simulink model "d2kontur_d2"  (R2014b)
settings: Solver=ode3  SolverMode=SingleTasking  StartTime=0.0  StopTime=10.0  RelTol=1e-3
PreLoadFcn:
  | waijung.modelPreload; % Required for working with Waijung Blockset. Do not remove.
undefined symbols (not defined in the file): FiO2, HCLK, HSEOSC, Link, LQFP100, ST, STM32F407VE
libraries: simulink_extras x8, stm32f4_io_lib x2, stm32f4_adc_lib x1, stm32f4_device_config_lib x1
(part 2 of 2)

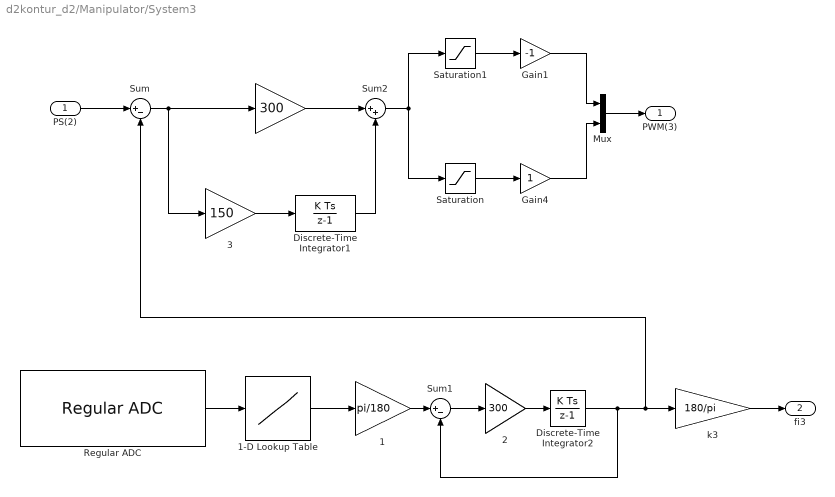
== system d2kontur_d2/Manipulator/System3 ==
  PS(2) : Inport
  " " : Gain  Gain=300
  " 1" : Gain  Gain=pi/180
  " 2" : Gain  Gain=300
  " 3" : Gain  Gain=150
  1-D Lookup Table : Lookup_n-D  NumberOfTableDimensions=1  BreakpointsForDimension1=[0 645 1470 2290 3115]  Table=[-180 -90 0 90 180]  InternalRulePriority=Speed  RndMeth=Simplest  InputSameDT=on
  Discrete-Time Integrator1 : DiscreteIntegrator  SampleTime=0.001  LimitOutput=on  UpperSaturationLimit=50  LowerSaturationLimit=-50
  Discrete-Time Integrator2 : DiscreteIntegrator  SampleTime=0.001
  Gain1 : Gain  Gain=-1  OutDataTypeStr=double
  Gain4 : Gain  OutDataTypeStr=double
  Mux : Mux  Inputs=2
  Regular ADC : stm32f4_adc_lib/Regular ADC  adcmodule=1  outputdatatype=Double  prescaler=2  prescalerstr=ADC_Prescaler_Div2  chsamplingtime=Auto  chsamplingtimestr=ADC_SampleTime_480Cycles  read_an0=off  read_an1=off  read_an2=off  read_an3=off  read_an4=off  read_an5=off  read_an6=off  read_an7=off  read_an8=off  read_an9=off  read_an10=off  read_an11=on  read_an12=off  read_an13=off  read_an14=off  read_an15=off  read_an16=off  read_an17=off  read_an18=off  pinstr=GPIO_Pin_11  usedpinarray="[0  0  0  0  0  0  0  0  0  0  0  1  0  0  0  0  0  0  0]"  usedportidarray=[2]  usedpinidarray=[1]  usedpinidcount=1  sampletime=0.001  blockid=ManipulatorSystem3RegularADC  enablecustomportlabel=off  cinputportlabel=0  coutputportlabel=Out1, Out2
  Saturation : Saturate  UpperLimit=80  LowerLimit=0  SampleTime=0.001
  Saturation1 : Saturate  UpperLimit=0  LowerLimit=-80  SampleTime=0.001
  Sum : Sum  Inputs=|+-
  Sum1 : Sum  Inputs=|+-
  Sum2 : Sum  Inputs=|++
  k3 : Gain  Gain=180/pi
  PWM(3) : Outport
  fi3 : Outport  Port=2
  wires:
  Saturation1/1 -> Gain1/1
  Saturation/1 -> Gain4/1
  PS(2)/1 -> Sum/1
  Gain1/1 -> Mux/1
  Gain4/1 -> Mux/2
  1-D Lookup Table/1 -> " 1"/1
  Mux/1 -> PWM(3)/1
  Sum2/1 -> Saturation/1, Saturation1/1
  Sum/1 -> " 3"/1, " "/1
  " 1"/1 -> Sum1/1
  Discrete-Time Integrator2/1 -> k3/1, Sum/2, Sum1/2
  Discrete-Time Integrator1/1 -> Sum2/2
  Regular ADC/1 -> 1-D Lookup Table/1
  " "/1 -> Sum2/1
  " 3"/1 -> Discrete-Time Integrator1/1
  Sum1/1 -> " 2"/1
  " 2"/1 -> Discrete-Time Integrator2/1
  k3/1 -> fi3/1

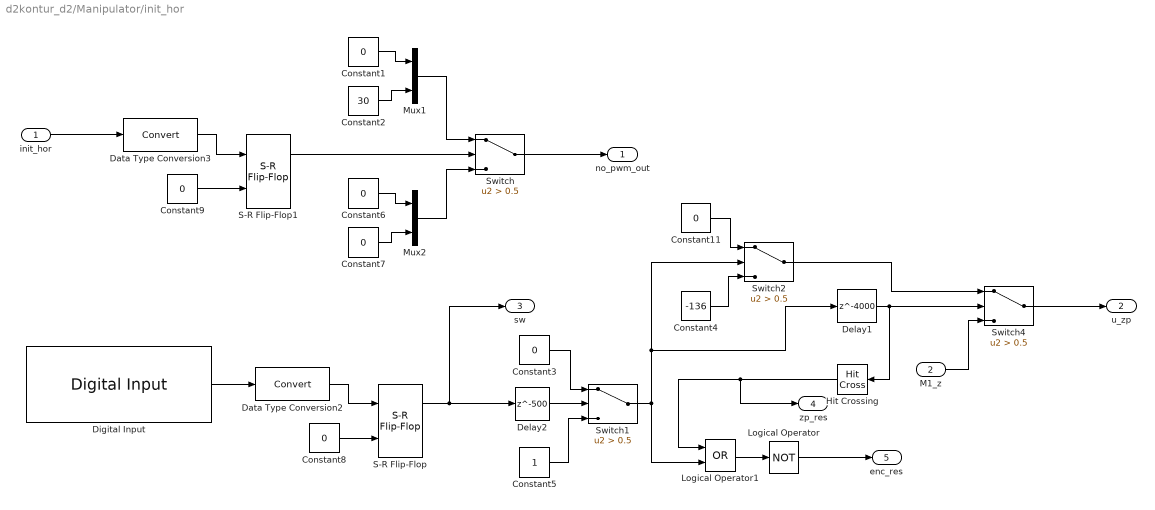
== system d2kontur_d2/Manipulator/init_hor ==
  init_hor : Inport
  M1_z : Inport  Port=2
  Constant{1,3,6..7,11} (5 alike) : Constant  Value=0
  Constant2 : Constant  Value=30
  Constant4 : Constant  Value=-136
  Constant5 : Constant
  Constant8 : Constant  Value=0  OutDataTypeStr=boolean
  Constant9 : Constant  Value=0  OutDataTypeStr=boolean
  Data Type Conversion2 : DataTypeConversion
  Data Type Conversion3 : DataTypeConversion
  Delay1 : Delay  DelayLength=4000
  Delay2 : Delay  DelayLength=500
  Digital Input : stm32f4_io_lib/Digital Input  port=B  speed=100  porttype=None  porttypestr=NOPULL  use_pin0=off  use_pin1=off  use_pin2=off  use_pin3=on  use_pin4=off  use_pin5=off  use_pin6=off  use_pin7=off  use_pin8=off  use_pin9=off  use_pin10=off  use_pin11=off  use_pin12=off  use_pin13=off  use_pin14=off  use_pin15=off  pinstr=GPIO_Pin_3  usedpinarray="[0  0  0  1  0  0  0  0  0  0  0  0  0  0  0  0]"  bitbandingstr="#define Manipulatorinit_horDigitalInput_B3 Peripheral_BB(GPIOB->IDR, 3)  /* Output pin */"  sampletime=0.001  sampletimestr=-1  blockid=Manipulatorinit_horDigitalInput  enablecustomportlabel=off  glabalinit=off  cinputportlabel=In1, In2  coutputportlabel=Out1, Out2
  Hit Crossing : HitCross  HitCrossingOffset=0.5  HitCrossingDirection=falling
  Logical Operator : Logic  Operator=NOT  AllPortsSameDT=off  OutDataTypeStr=boolean
  Logical Operator1 : Logic  Operator=OR  AllPortsSameDT=off  OutDataTypeStr=boolean
  Mux1 : Mux  Inputs=2
  Mux2 : Mux  Inputs=2
  S-R Flip-Flop : simulink_extras/Flip Flops/S-R Flip-Flop  initial_condition=0
  S-R Flip-Flop1 : simulink_extras/Flip Flops/S-R Flip-Flop  initial_condition=0
  Switch{,1..2,4} (4 alike) : Switch  Criteria=u2 > Threshold  Threshold=0.5
  no_pwm_out : Outport
  u_zp : Outport  Port=2
  sw : Outport  Port=3
  zp_res : Outport  Port=4
  enc_res : Outport  Port=5
  wires:
  init_hor/1 -> Data Type Conversion3/1
  Constant5/1 -> Switch1/3
  S-R Flip-Flop1/1 -> Switch/2
  Switch2/1 -> Switch4/1
  Data Type Conversion3/1 -> S-R Flip-Flop1/1
  Constant9/1 -> S-R Flip-Flop1/2
  S-R Flip-Flop/1 -> sw/1, Delay2/1
  Switch4/1 -> u_zp/1
  Switch/1 -> no_pwm_out/1
  Digital Input/1 -> Data Type Conversion2/1
  Constant8/1 -> S-R Flip-Flop/2
  Data Type Conversion2/1 -> S-R Flip-Flop/1
  Mux2/1 -> Switch/3
  Mux1/1 -> Switch/1
  Hit Crossing/1 -> zp_res/1, Logical Operator1/1
  M1_z/1 -> Switch4/3
  Logical Operator/1 -> enc_res/1
  Delay1/1 -> Switch4/2, Hit Crossing/1
  Switch1/1 -> Logical Operator1/2, Delay1/1, Switch2/2
  Delay2/1 -> Switch1/2
  Logical Operator1/1 -> Logical Operator/1
  Constant1/1 -> Mux1/1
  Constant2/1 -> Mux1/2
  Constant6/1 -> Mux2/1
  Constant7/1 -> Mux2/2
  Constant3/1 -> Switch1/1
  Constant4/1 -> Switch2/3
  Constant11/1 -> Switch2/1

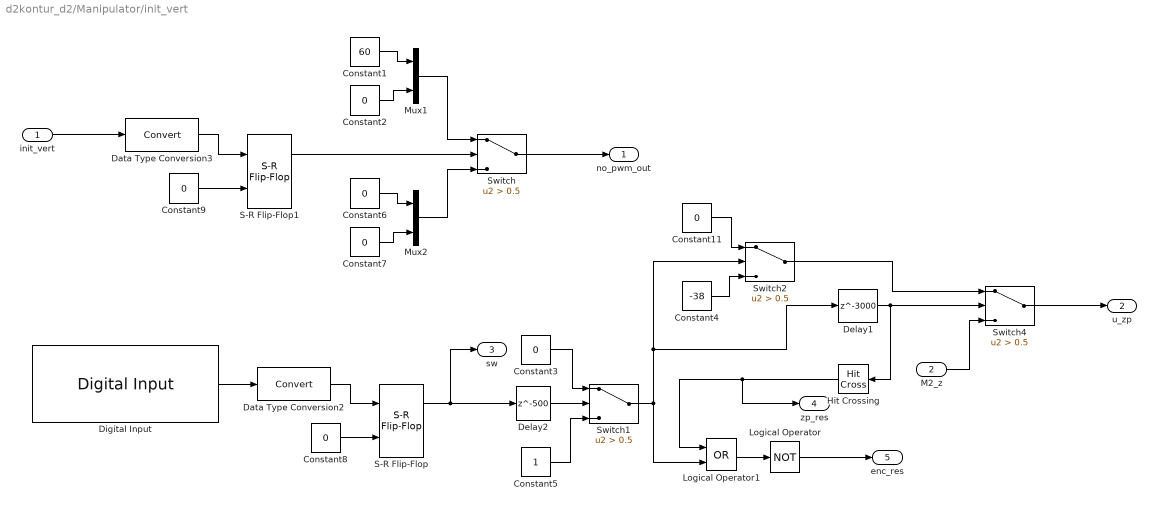
== system d2kontur_d2/Manipulator/init_vert ==
  init_vert : Inport
  M2_z : Inport  Port=2
  Constant1 : Constant  Value=60
  Constant{2..3,6..7,11} (5 alike) : Constant  Value=0
  Constant4 : Constant  Value=-38
  Constant5 : Constant
  Constant8 : Constant  Value=0  OutDataTypeStr=boolean
  Constant9 : Constant  Value=0  OutDataTypeStr=boolean
  Data Type Conversion2 : DataTypeConversion
  Data Type Conversion3 : DataTypeConversion
  Delay1 : Delay  DelayLength=3000
  Delay2 : Delay  DelayLength=500
  Digital Input : stm32f4_io_lib/Digital Input  port=D  speed=100  porttype=None  porttypestr=NOPULL  use_pin0=on  use_pin1=off  use_pin2=off  use_pin3=off  use_pin4=off  use_pin5=off  use_pin6=off  use_pin7=off  use_pin8=off  use_pin9=off  use_pin10=off  use_pin11=off  use_pin12=off  use_pin13=off  use_pin14=off  use_pin15=off  pinstr=GPIO_Pin_0  usedpinarray="[1  0  0  0  0  0  0  0  0  0  0  0  0  0  0  0]"  bitbandingstr="#define Manipulatorinit_vertDigitalInput_D0 Peripheral_BB(GPIOD->IDR, 0)  /* Output pin */"  sampletime=0.001  sampletimestr=-1  blockid=Manipulatorinit_vertDigitalInput  enablecustomportlabel=off  glabalinit=off  cinputportlabel=In1, In2  coutputportlabel=Out1, Out2
  Hit Crossing : HitCross  HitCrossingOffset=0.5  HitCrossingDirection=falling
  Logical Operator : Logic  Operator=NOT  AllPortsSameDT=off  OutDataTypeStr=boolean
  Logical Operator1 : Logic  Operator=OR  AllPortsSameDT=off  OutDataTypeStr=boolean
  Mux1 : Mux  Inputs=2
  Mux2 : Mux  Inputs=2
  S-R Flip-Flop : simulink_extras/Flip Flops/S-R Flip-Flop  initial_condition=0
  S-R Flip-Flop1 : simulink_extras/Flip Flops/S-R Flip-Flop  initial_condition=0
  Switch{,1..2,4} (4 alike) : Switch  Criteria=u2 > Threshold  Threshold=0.5
  no_pwm_out : Outport
  u_zp : Outport  Port=2
  sw : Outport  Port=3
  zp_res : Outport  Port=4
  enc_res : Outport  Port=5
  wires:
  Constant11/1 -> Switch2/1
  Constant3/1 -> Switch1/1
  Constant7/1 -> Mux2/2
  Constant6/1 -> Mux2/1
  Constant2/1 -> Mux1/2
  Constant1/1 -> Mux1/1
  Logical Operator1/1 -> Logical Operator/1
  Delay2/1 -> Switch1/2
  Switch1/1 -> Switch2/2, Delay1/1, Logical Operator1/2
  Delay1/1 -> Hit Crossing/1, Switch4/2
  Logical Operator/1 -> enc_res/1
  M2_z/1 -> Switch4/3
  Hit Crossing/1 -> Logical Operator1/1, zp_res/1
  Mux1/1 -> Switch/1
  Mux2/1 -> Switch/3
  Data Type Conversion2/1 -> S-R Flip-Flop/1
  Constant8/1 -> S-R Flip-Flop/2
  Digital Input/1 -> Data Type Conversion2/1
  Switch/1 -> no_pwm_out/1
  Switch4/1 -> u_zp/1
  S-R Flip-Flop/1 -> Delay2/1, sw/1
  Constant9/1 -> S-R Flip-Flop1/2
  Data Type Conversion3/1 -> S-R Flip-Flop1/1
  Switch2/1 -> Switch4/1
  S-R Flip-Flop1/1 -> Switch/2
  Constant5/1 -> Switch1/3
  init_vert/1 -> Data Type Conversion3/1
  Constant4/1 -> Switch2/3

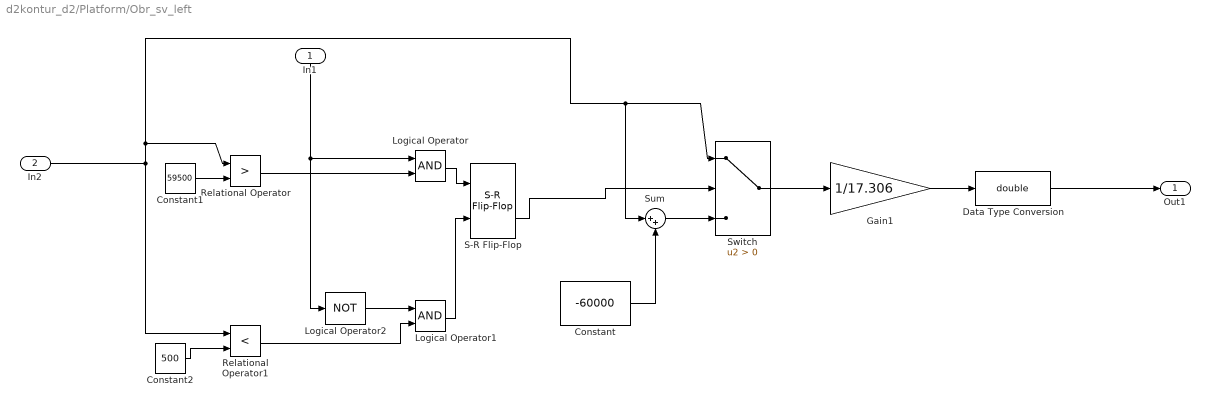
== system d2kontur_d2/Platform/Obr_sv_left ==
  In1 : Inport
  In2 : Inport  Port=2
  Constant : Constant  Value=-60000
  Constant1 : Constant  Value=59500
  Constant2 : Constant  Value=500
  Data Type Conversion : DataTypeConversion  OutDataTypeStr=double
  Gain1 : Gain  Gain=1/17.306
  Logical Operator : Logic  AllPortsSameDT=off  OutDataTypeStr=boolean
  Logical Operator1 : Logic  AllPortsSameDT=off  OutDataTypeStr=boolean
  Logical Operator2 : Logic  Operator=NOT  AllPortsSameDT=off  OutDataTypeStr=boolean
  Relational Operator : RelationalOperator  Operator=>  OutDataTypeStr=boolean
  Relational Operator1 : RelationalOperator  Operator=<  OutDataTypeStr=boolean
  S-R Flip-Flop : simulink_extras/Flip Flops/S-R Flip-Flop  initial_condition=0
  Sum : Sum  Inputs=|++
  Switch : Switch  Criteria=u2 > Threshold
  Out1 : Outport
  wires:
  Constant/1 -> Sum/2
  Relational Operator/1 -> Logical Operator/2
  Logical Operator/1 -> S-R Flip-Flop/1
  Relational Operator1/1 -> Logical Operator1/2
  Logical Operator1/1 -> S-R Flip-Flop/2
  In2/1 -> Switch/1, Sum/1, Relational Operator/1, Relational Operator1/1
  Sum/1 -> Switch/3
  Constant1/1 -> Relational Operator/2
  Constant2/1 -> Relational Operator1/2
  S-R Flip-Flop/2 -> Switch/2
  In1/1 -> Logical Operator/1, Logical Operator2/1
  Logical Operator2/1 -> Logical Operator1/1
  Gain1/1 -> Data Type Conversion/1
  Switch/1 -> Gain1/1
  Data Type Conversion/1 -> Out1/1

== system d2kontur_d2/Platform/Obr_sv_right ==
  In1 : Inport
  In2 : Inport  Port=2
  Constant : Constant  Value=-60000
  Constant1 : Constant  Value=59500
  Constant2 : Constant  Value=500
  Data Type Conversion : DataTypeConversion  OutDataTypeStr=double
  Gain1 : Gain  Gain=1/17.306
  Logical Operator : Logic  AllPortsSameDT=off  OutDataTypeStr=boolean
  Logical Operator1 : Logic  AllPortsSameDT=off  OutDataTypeStr=boolean
  Logical Operator2 : Logic  Operator=NOT  AllPortsSameDT=off  OutDataTypeStr=boolean
  Relational Operator : RelationalOperator  Operator=>  OutDataTypeStr=boolean
  Relational Operator1 : RelationalOperator  Operator=<  OutDataTypeStr=boolean
  S-R Flip-Flop : simulink_extras/Flip Flops/S-R Flip-Flop  initial_condition=0
  Sum : Sum  Inputs=|++
  Switch : Switch  Criteria=u2 > Threshold
  Out1 : Outport
  wires:
  Logical Operator2/1 -> Logical Operator1/1
  In1/1 -> Logical Operator2/1, Logical Operator/1
  S-R Flip-Flop/2 -> Switch/2
  Constant2/1 -> Relational Operator1/2
  Constant1/1 -> Relational Operator/2
  Sum/1 -> Switch/3
  In2/1 -> Relational Operator1/1, Relational Operator/1, Sum/1, Switch/1
  Logical Operator1/1 -> S-R Flip-Flop/2
  Relational Operator1/1 -> Logical Operator1/2
  Logical Operator/1 -> S-R Flip-Flop/1
  Relational Operator/1 -> Logical Operator/2
  Constant/1 -> Sum/2
  Gain1/1 -> Data Type Conversion/1
  Switch/1 -> Gain1/1
  Data Type Conversion/1 -> Out1/1

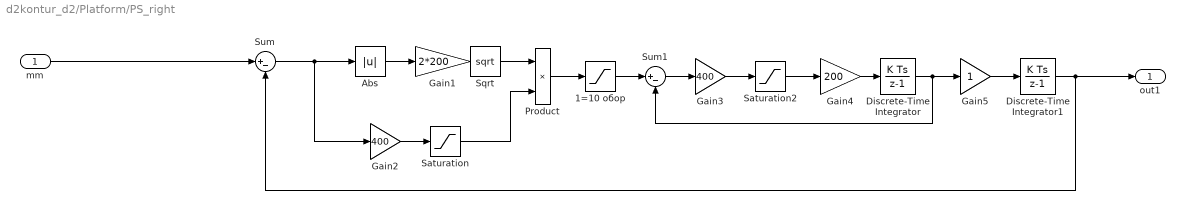
== system d2kontur_d2/Platform/PS_right  ==
  mm : Inport
  1=10 обор : Saturate  UpperLimit=200  LowerLimit=-200
  Abs : Abs
  Discrete-Time Integrator : DiscreteIntegrator  SampleTime=0.001
  Discrete-Time Integrator1 : DiscreteIntegrator  SampleTime=0.001
  Gain1 : Gain  Gain=2*200
  Gain2 : Gain  Gain=400
  Gain3 : Gain  Gain=400
  Gain4 : Gain  Gain=200
  Gain5 : Gain
  Product : Product
  Saturation : Saturate  UpperLimit=1  LowerLimit=-1
  Saturation2 : Saturate  UpperLimit=1  LowerLimit=-1
  Sqrt : Sqrt  SaturateOnIntegerOverflow=on
  Sum : Sum  Inputs=|+-
  Sum1 : Sum  Inputs=|+-
  "out1 " : Outport
  wires:
  mm/1 -> Sum/1
  Abs/1 -> Gain1/1
  Sum/1 -> Gain2/1, Abs/1
  Gain1/1 -> Sqrt/1
  Sqrt/1 -> Product/1
  Gain3/1 -> Saturation2/1
  1=10 обор/1 -> Sum1/1
  Saturation/1 -> Product/2
  Discrete-Time Integrator1/1 -> "out1 "/1, Sum/2
  Product/1 -> 1=10 обор/1
  Gain5/1 -> Discrete-Time Integrator1/1
  Sum1/1 -> Gain3/1
  Gain2/1 -> Saturation/1
  Discrete-Time Integrator/1 -> Gain5/1, Sum1/2
  Saturation2/1 -> Gain4/1
  Gain4/1 -> Discrete-Time Integrator/1

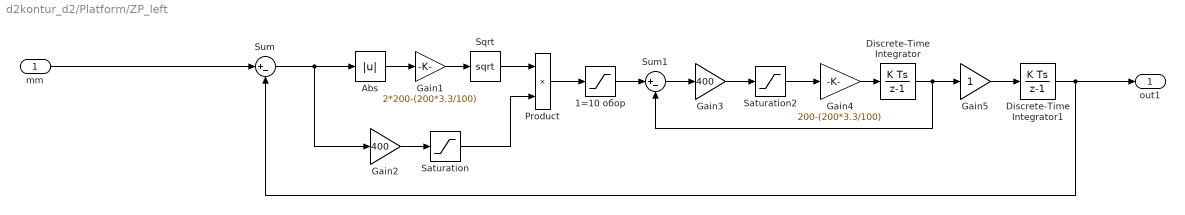
== system d2kontur_d2/Platform/ZP_left ==
  mm : Inport
  1=10 обор : Saturate  UpperLimit=200-(200*3.3/100)  LowerLimit=-(200-(200*3.3/100))
  Abs : Abs
  Discrete-Time Integrator : DiscreteIntegrator  SampleTime=0.001
  Discrete-Time Integrator1 : DiscreteIntegrator  SampleTime=0.001
  Gain1 : Gain  Gain=2*200-(200*3.3/100)
  Gain2 : Gain  Gain=400
  Gain3 : Gain  Gain=400
  Gain4 : Gain  Gain=200-(200*3.3/100)
  Gain5 : Gain
  Product : Product
  Saturation : Saturate  UpperLimit=1  LowerLimit=-1
  Saturation2 : Saturate  UpperLimit=1  LowerLimit=-1
  Sqrt : Sqrt  SaturateOnIntegerOverflow=on
  Sum : Sum  Inputs=|+-
  Sum1 : Sum  Inputs=|+-
  "out1 " : Outport
  wires:
  Gain4/1 -> Discrete-Time Integrator/1
  Saturation2/1 -> Gain4/1
  Discrete-Time Integrator/1 -> Sum1/2, Gain5/1
  Gain2/1 -> Saturation/1
  Sum1/1 -> Gain3/1
  Gain5/1 -> Discrete-Time Integrator1/1
  Product/1 -> 1=10 обор/1
  Discrete-Time Integrator1/1 -> Sum/2, "out1 "/1
  Saturation/1 -> Product/2
  1=10 обор/1 -> Sum1/1
  Gain3/1 -> Saturation2/1
  Sqrt/1 -> Product/1
  Gain1/1 -> Sqrt/1
  Sum/1 -> Abs/1, Gain2/1
  Abs/1 -> Gain1/1
  mm/1 -> Sum/1

== system d2kontur_d2/Platform/left ==
  Zadanie : Inport
  Obr_sv : Inport  Port=2
  Gain1 : Gain  Gain=-1
  Gain5 : Gain  Gain=10
  Saturation1 : Saturate  UpperLimit=100  LowerLimit=0
  Saturation4 : Saturate  UpperLimit=0  LowerLimit=-100
  Sum : Sum  Inputs=|+-
  Out1 : Outport
  Out2 : Outport  Port=2
  wires:
  Gain1/1 -> Out1/1
  Saturation1/1 -> Out2/1
  Saturation4/1 -> Gain1/1
  Zadanie/1 -> Sum/1
  Obr_sv/1 -> Sum/2
  Gain5/1 -> Saturation4/1, Saturation1/1
  Sum/1 -> Gain5/1

== system d2kontur_d2/Platform/right ==
  Zadanie : Inport
  Obr_sv : Inport  Port=2
  Gain1 : Gain  Gain=-1
  Gain4 : Gain  Gain=-1
  Gain5 : Gain  Gain=10
  Saturation1 : Saturate  UpperLimit=100  LowerLimit=0
  Saturation4 : Saturate  UpperLimit=0  LowerLimit=-100
  Sum : Sum  Inputs=|+-
  Out1 : Outport
  Out2 : Outport  Port=2
  wires:
  Obr_sv/1 -> Sum/2
  Zadanie/1 -> Gain4/1
  Saturation4/1 -> Gain1/1
  Saturation1/1 -> Out2/1
  Gain1/1 -> Out1/1
  Gain5/1 -> Saturation4/1, Saturation1/1
  Sum/1 -> Gain5/1
  Gain4/1 -> Sum/1

== system d2kontur_d2/Signal_generation/SW1 ==
  ind2 : Inport
  ind1 : Inport  Port=2
  sravn : Inport  Port=3
  "Obr_sv " : Inport  Port=4
  Relational Operator : RelationalOperator  Operator===  OutDataTypeStr=boolean
  Switch3 : Switch  Criteria=u2 > Threshold  Threshold=0.5
  M1 : Outport
  wires:
  ind1/1 -> Relational Operator/1
  Switch3/1 -> M1/1
  sravn/1 -> Relational Operator/2
  "Obr_sv "/1 -> Switch3/3
  ind2/1 -> Switch3/1
  Relational Operator/1 -> Switch3/2

== system d2kontur_d2/Signal_generation/SW2 ==
  ind2 : Inport
  ind1 : Inport  Port=2
  sravn : Inport  Port=3
  "Obr_sv " : Inport  Port=4
  Relational Operator : RelationalOperator  Operator===  OutDataTypeStr=boolean
  Switch3 : Switch  Criteria=u2 > Threshold  Threshold=0.5
  M2 : Outport
  wires:
  Relational Operator/1 -> Switch3/2
  ind2/1 -> Switch3/1
  "Obr_sv "/1 -> Switch3/3
  sravn/1 -> Relational Operator/2
  Switch3/1 -> M2/1
  ind1/1 -> Relational Operator/1

== system d2kontur_d2/Signal_generation/SW3 ==
  ind2 : Inport
  ind1 : Inport  Port=2
  sravn : Inport  Port=3
  "Obr_sv " : Inport  Port=4
  Relational Operator : RelationalOperator  Operator===  OutDataTypeStr=boolean
  Switch3 : Switch  Criteria=u2 > Threshold  Threshold=0.5
  M3 : Outport
  wires:
  ind1/1 -> Relational Operator/1
  Switch3/1 -> M3/1
  sravn/1 -> Relational Operator/2
  "Obr_sv "/1 -> Switch3/3
  ind2/1 -> Switch3/1
  Relational Operator/1 -> Switch3/2

== system d2kontur_d2/Signal_generation/SWT ==
  ind2 : Inport
  ind1 : Inport  Port=2
  sravn : Inport  Port=3
  "Obr_sv " : Inport  Port=4
  Relational Operator : RelationalOperator  Operator===  OutDataTypeStr=boolean
  Switch3 : Switch  Criteria=u2 > Threshold  Threshold=0.5
  Platform : Outport
  wires:
  Relational Operator/1 -> Switch3/2
  ind2/1 -> Switch3/1
  "Obr_sv "/1 -> Switch3/3
  sravn/1 -> Relational Operator/2
  Switch3/1 -> Platform/1
  ind1/1 -> Relational Operator/1

== system d2kontur_d2/Manipulator/System1/PositionFeedback ==
  Enable : EnablePort
  Data Type Conversion1 : DataTypeConversion  OutDataTypeStr=double
  Data Type Conversion2 : DataTypeConversion  OutDataTypeStr=double
  Encoder Read1 : S-Function  FunctionName=stm32f4_encoderread  Parameters=sampletime,sampletimestr,blockid,timer,apb,portstr,pinstr,pinmat,chmat,filterstr,filter,factor,rstcnt,ppr  EnableBusSupport=off  mask(stm32f4_encoderread){timer=3, ch1=A6, ch2=B5, ppr=10000, rstcnt=off, filterstr=No filter; sampling is done at fDTS, sampletime=0.001, sampletimestr=-1, blockid=ManipulatorSystem1PositionFeedbackEncoderRead1, absresetinput=off, portpinstr=A6,B5, portstr=["A","B"], pinstr=["GPIO_Pin_6","GPIO_Pin_5"], pinmat=[1 6;1 5], chmat=[1  2], apb=1, filter=0, factor=4}
      mask prompts: ch1 "Channel A Input Pin"; ch2 "Channel B Input Pin"; ppr "PPR (Number of pulses generated per revolution)"; rstcnt "Reset counter after every counter read"; filterstr "Built-in Input Capture Filter"; sampletime "Sample time (sec)"; sampletimestr "Compiled sample time (sec) in string"; absresetinput "Enable absolute position reset input signal"; portpinstr "Port pin string"; portstr "Port string"; pinstr "Pin string"; pinmat "Pin matrix"; chmat "Channel order"; filter "Filter ID"
      mask help:
      | The output Direction (uint32) is the direction of rotation either 0 or 1.
      |
      | The output Position (count) (uint32) is the count of number of edges of the encoder output signals from either channel A and B. The decoder is set to count at every rising and falling edge of both channel A and B (4x) or (x2) for one channel. For example, if an encoder has 180 pulses per revolution (PPS) and two channels are selected, the maximum count is 720 per revolution (4x180 = 720), i.e. from 0 to 719.
      mask init:
      | stm32f4_encoderread_callback('init');
      mask Help: web(fullfile(waijungdocroot,'stm32f4_encoderread.htm'),'-browser')
      mask TypeOptions timer: 1 | 2 | 3 | 4 | 5 | 8
      mask Callback timer: stm32f4_encoderread_callback('timer');
      mask TypeOptions ch1: Not available - Do not use | A6 | C6 | B4
      mask Callback ch1: stm32f4_encoderread_callback('chA');
      mask TypeOptions ch2: Not available - Do not use | A7 | C7 | B5
      mask Callback ch2: stm32f4_encoderread_callback('chB');
      mask Callback ppr: stm32f4_encoderread_callback('ppr');
      mask Callback rstcnt: stm32f4_encoderread_callback('rstcnt');
      mask TypeOptions filterstr: No filter; sampling is done at fDTS | fSAMPLING=fCK_INT; N=2 | fSAMPLING=fCK_INT; N=4 | fSAMPLING=fCK_INT; N=8 | fSAMPLING=fDTS/2; N=6 | fSAMPLING=fDTS/2; N=8 | fSAMPLING=fDTS/4; N=6 | fSAMPLING=fDTS/4; N=8 | fSAMPLING=fDTS/8; N=6 | fSAMPLING=fDTS/8; N=8 | fSAMPLING=fDTS/16; N=5 | fSAMPLING=fDTS/16; N=6 | fSAMPLING=fDTS/16; N=8 | fSAMPLING=fDTS/32; N=5 | fSAMPLING=fDTS/32; N=6 | fSAMPLING=fDTS/32; N=8
      mask Callback filterstr: stm32f4_encoderread_callback('filterstr');
      mask Callback sampletimestr: stm32f4_encoderread_callback('sampletimestr');
      mask Callback blockid: stm32f4_encoderread_callback('blockid');
      mask Display: text(0.05, 0.5, 'Timer: 3\nInput pins [CH_A, CH_B]: [A6,B5]\nRST Counter: No\nTs (sec): -1','ver','middle','hor','left');port_label('output', 1, 'Direction');port_label('output', 2, 'Position (count)')
  To_Bipolar : Subsystem
  To_radians : Gain  Gain=pi/48.8/180
  ps_rad : Outport
  wires:
  To_Bipolar/1(Out1) -> To_radians/1
  Encoder Read1/2 -> Data Type Conversion1/1
  Encoder Read1/1 -> Data Type Conversion2/1
  Data Type Conversion2/1 -> To_Bipolar/1(In1)
  To_radians/1 -> ps_rad/1
  Data Type Conversion1/1 -> To_Bipolar/2(In2)

== system d2kontur_d2/Manipulator/System2/Subsystem ==
  Enable : EnablePort
  Data Type Conversion1 : DataTypeConversion  OutDataTypeStr=double
  Data Type Conversion2 : DataTypeConversion  OutDataTypeStr=double
  Encoder Read : S-Function  FunctionName=stm32f4_encoderread  Parameters=sampletime,sampletimestr,blockid,timer,apb,portstr,pinstr,pinmat,chmat,filterstr,filter,factor,rstcnt,ppr  EnableBusSupport=off  mask(stm32f4_encoderread){timer=4, ch1=B6, ch2=B7, ppr=27034, rstcnt=off, filterstr=No filter; sampling is done at fDTS, sampletime=0.001, sampletimestr=-1, blockid=ManipulatorSystem2SubsystemEncoderRead, absresetinput=off, portpinstr=B6,B7, portstr=["B"], pinstr=["GPIO_Pin_6 | GPIO_Pin_7"], pinmat=[2 6 7], chmat=[1  2], apb=1, filter=0, factor=4}
      mask prompts: ch1 "Channel A Input Pin"; ch2 "Channel B Input Pin"; ppr "PPR (Number of pulses generated per revolution)"; rstcnt "Reset counter after every counter read"; filterstr "Built-in Input Capture Filter"; sampletime "Sample time (sec)"; sampletimestr "Compiled sample time (sec) in string"; absresetinput "Enable absolute position reset input signal"; portpinstr "Port pin string"; portstr "Port string"; pinstr "Pin string"; pinmat "Pin matrix"; chmat "Channel order"; filter "Filter ID"
      mask help:
      | The output Direction (uint32) is the direction of rotation either 0 or 1.
      |
      | The output Position (count) (uint32) is the count of number of edges of the encoder output signals from either channel A and B. The decoder is set to count at every rising and falling edge of both channel A and B (4x) or (x2) for one channel. For example, if an encoder has 180 pulses per revolution (PPS) and two channels are selected, the maximum count is 720 per revolution (4x180 = 720), i.e. from 0 to 719.
      mask init:
      | stm32f4_encoderread_callback('init');
      mask Help: web(fullfile(waijungdocroot,'stm32f4_encoderread.htm'),'-browser')
      mask TypeOptions timer: 1 | 2 | 3 | 4 | 5 | 8
      mask Callback timer: stm32f4_encoderread_callback('timer');
      mask TypeOptions ch1: Not available - Do not use | D12 | B6
      mask Callback ch1: stm32f4_encoderread_callback('chA');
      mask TypeOptions ch2: Not available - Do not use | D13 | B7
      mask Callback ch2: stm32f4_encoderread_callback('chB');
      mask Callback ppr: stm32f4_encoderread_callback('ppr');
      mask Callback rstcnt: stm32f4_encoderread_callback('rstcnt');
      mask TypeOptions filterstr: No filter; sampling is done at fDTS | fSAMPLING=fCK_INT; N=2 | fSAMPLING=fCK_INT; N=4 | fSAMPLING=fCK_INT; N=8 | fSAMPLING=fDTS/2; N=6 | fSAMPLING=fDTS/2; N=8 | fSAMPLING=fDTS/4; N=6 | fSAMPLING=fDTS/4; N=8 | fSAMPLING=fDTS/8; N=6 | fSAMPLING=fDTS/8; N=8 | fSAMPLING=fDTS/16; N=5 | fSAMPLING=fDTS/16; N=6 | fSAMPLING=fDTS/16; N=8 | fSAMPLING=fDTS/32; N=5 | fSAMPLING=fDTS/32; N=6 | fSAMPLING=fDTS/32; N=8
      mask Callback filterstr: stm32f4_encoderread_callback('filterstr');
      mask Callback sampletimestr: stm32f4_encoderread_callback('sampletimestr');
      mask Callback blockid: stm32f4_encoderread_callback('blockid');
      mask Display: text(0.05, 0.5, 'Timer: 4\nInput pins [CH_A, CH_B]: [B6,B7]\nRST Counter: No\nTs (sec): -1','ver','middle','hor','left');port_label('output', 1, 'Direction');port_label('output', 2, 'Position (count)')
  Subsystem2 : Subsystem
  перевод в радианы : Gain  Gain=pi/73/180
  oc_rad : Outport
  wires:
  Encoder Read/2 -> Data Type Conversion1/1
  Data Type Conversion1/1 -> Subsystem2/2(In2)
  Subsystem2/1(Out1) -> перевод в радианы/1
  перевод в радианы/1 -> oc_rad/1
  Data Type Conversion2/1 -> Subsystem2/1(In1)
  Encoder Read/1 -> Data Type Conversion2/1

== system d2kontur_d2/Manipulator/System1/PositionFeedback/To_Bipolar ==
  In1 : Inport
  In2 : Inport  Port=2
  Constant : Constant  Value=-40000
  Constant1 : Constant  Value=39500
  Constant2 : Constant  Value=500
  Logical Operator : Logic  AllPortsSameDT=off  OutDataTypeStr=boolean
  Logical Operator1 : Logic  AllPortsSameDT=off  OutDataTypeStr=boolean
  Logical Operator2 : Logic  Operator=NOT  AllPortsSameDT=off  OutDataTypeStr=boolean
  Relational Operator : RelationalOperator  Operator=>  OutDataTypeStr=boolean
  Relational Operator1 : RelationalOperator  Operator=<  OutDataTypeStr=boolean
  S-R Flip-Flop : simulink_extras/Flip Flops/S-R Flip-Flop  initial_condition=0
  Sum : Sum  Inputs=|++
  Switch : Switch  Criteria=u2 > Threshold
  Out1 : Outport
  wires:
  Logical Operator2/1 -> Logical Operator1/1
  In1/1 -> Logical Operator2/1, Logical Operator/1
  S-R Flip-Flop/2 -> Switch/2
  Constant2/1 -> Relational Operator1/2
  Constant1/1 -> Relational Operator/2
  Sum/1 -> Switch/3
  Switch/1 -> Out1/1
  In2/1 -> Relational Operator1/1, Relational Operator/1, Sum/1, Switch/1
  Logical Operator1/1 -> S-R Flip-Flop/2
  Relational Operator1/1 -> Logical Operator1/2
  Logical Operator/1 -> S-R Flip-Flop/1
  Relational Operator/1 -> Logical Operator/2
  Constant/1 -> Sum/2

== system d2kontur_d2/Manipulator/System2/Subsystem/Subsystem2 ==
  In1 : Inport
  In2 : Inport  Port=2
  Constant : Constant  Value=-27034-15559
  Constant1 : Constant  Value=42000
  Constant2 : Constant  Value=100
  Logical Operator : Logic  AllPortsSameDT=off  OutDataTypeStr=boolean
  Logical Operator1 : Logic  AllPortsSameDT=off  OutDataTypeStr=boolean
  Logical Operator2 : Logic  Operator=NOT  AllPortsSameDT=off  OutDataTypeStr=boolean
  Relational Operator : RelationalOperator  Operator=>  OutDataTypeStr=boolean
  Relational Operator1 : RelationalOperator  Operator=<  OutDataTypeStr=boolean
  S-R Flip-Flop : simulink_extras/Flip Flops/S-R Flip-Flop  initial_condition=0
  Sum : Sum  Inputs=|++
  Switch : Switch  Criteria=u2 > Threshold
  Out1 : Outport
  wires:
  Logical Operator2/1 -> Logical Operator1/1
  In1/1 -> Logical Operator2/1, Logical Operator/1
  S-R Flip-Flop/2 -> Switch/2
  Constant2/1 -> Relational Operator1/2
  Constant1/1 -> Relational Operator/2
  Sum/1 -> Switch/3
  Switch/1 -> Out1/1
  In2/1 -> Relational Operator1/1, Relational Operator/1, Sum/1, Switch/1
  Logical Operator1/1 -> S-R Flip-Flop/2
  Relational Operator1/1 -> Logical Operator1/2
  Logical Operator/1 -> S-R Flip-Flop/1
  Relational Operator/1 -> Logical Operator/2
  Constant/1 -> Sum/2
